simulink model "ScriptDemo"  (R2022b)
settings: configuration reference "TmVcThermal_Configuration_sub" (kept outside this file)
undefined symbols (not defined in the file or in its folder): aaaa, bbbb, cTmComprCtrl_D_u8HvacFlowTable_db, cTmComprCtrl_D_u8HvacFlowTable_sw, cTmComprCtrl_n_i16ChillCmpIMax, cTmComprCtrl_n_i16ChillCmpIMin, cTmComprCtrl_n_i16ChillCmpIMin666, cTmComprCtrl_n_i16ChillCmpPMax, cTmComprCtrl_n_i16ChillCmpPMin, cTmComprCtrl_n_i16CmpChillCoolRpmKiMax, cTmComprCtrl_n_i16CmpChillCoolRpmKiMin, cTmComprCtrl_n_i16CmpChillCoolRpmKpMax, cTmComprCtrl_n_i16CmpChillCoolRpmKpMin, cTmComprCtrl_n_i16CmpCoolRpmKiMax, cTmComprCtrl_n_i16CmpCoolRpmKiMin, cTmComprCtrl_n_i16CmpCoolRpmKpMax, cTmComprCtrl_n_i16CmpCoolRpmKpMin, cTmComprCtrl_n_i16SM4CmpHeatKiMax, cTmComprCtrl_n_i16SM4CmpHeatKiMin, cTmComprCtrl_n_i16SM4CmpHeatKpMax, cTmComprCtrl_n_i16SM4CmpHeatKpMin, cTmComprCtrl_n_i16SM5CmpHeatKiMax, cTmComprCtrl_n_i16SM5CmpHeatKiMin, cTmComprCtrl_n_i16SM5CmpHeatKpMax, cTmComprCtrl_n_i16SM5CmpHeatKpMin, cTmComprCtrl_n_i16SM6CmpHeatKiMax, cTmComprCtrl_n_i16SM6CmpHeatKiMin, cTmComprCtrl_n_i16SM6CmpHeatKpMax, cTmComprCtrl_n_i16SM6CmpHeatKpMin, cTmComprCtrl_n_u16CmpMaxSpdFanFltLimt, cTmComprCtrl_n_u16CmpMaxSpdLoSidePFltLimt, cTmComprCtrl_n_u16CmpMaxSpdSensorFltLimt, cTmComprCtrl_n_u16CompMinRpm, cTmComprCtrl_n_u16CompRpmIncThres, cTmComprCtrl_t_u16BattCooltFFPeriod, cTmComprCtrl_t_u16BattCooltPIPeriod, cTmComprCtrl_t_u16CmpCoolFFPeriod, cTmComprCtrl_t_u16CmpCoolPIPeriod, cTmComprCtrl_t_u16CoolCmpChillFFPeriod, cTmComprCtrl_t_u16CoolCmpChillPIPeriod, cTmComprCtrl_t_u16SM4CmpHeatFFPeriod, cTmComprCtrl_t_u16SM4CmpHeatPIPeriod, cTmComprCtrl_t_u16SM5CmpHeatFFPeriod, cTmComprCtrl_t_u16SM5CmpHeatPIPeriod, cTmComprCtrl_t_u16SM6CmpHeatFFPeriod, cTmComprCtrl_t_u16SM6CmpHeatPIPeriod, cTmComprCtrl_Te_EvapClearInteg, cTmComprCtrl_Te_i16HpReqTempSaturoffset, cTmComprCtrl_Te_i16SatLpReplaceDiff, cTmComprCtrl_Te_i16SM3BatDiffStartEvapDecOffset, cTmComprCtrl_Te_i16SM3EvapLo, cTmComprCtrl_Te_i16SM3TBatDiffEntEvapDecOffset, cTmComprCtrl_Te_i16SM3TBatDiffEntEvapDecOffsetQuit, cTmComprCtrl_Te_s32ErrCmpChillPIContinueCoolH, cTmComprCtrl_Te_s32ErrCmpChillPIContinueCoolL, cTmComprCtrl_Te_s32ErrCmpPIContinueChillH, cTmComprCtrl_Te_s32ErrCmpPIContinueChillL, cTmComprCtrl_Te_s32ErrCmpPIContinueCoolH, cTmComprCtrl_Te_s32ErrCmpPIContinueCoolL, cTmComprCtrl_Te_s32ErrCmpPIContinueHeatH ... (+398)
libraries: simulink x846, PCMULib x711, simulink_need_slupdate x4
(part 8 of 49)

== system ScriptDemo/Create/creatTmBaseArch/Before ==

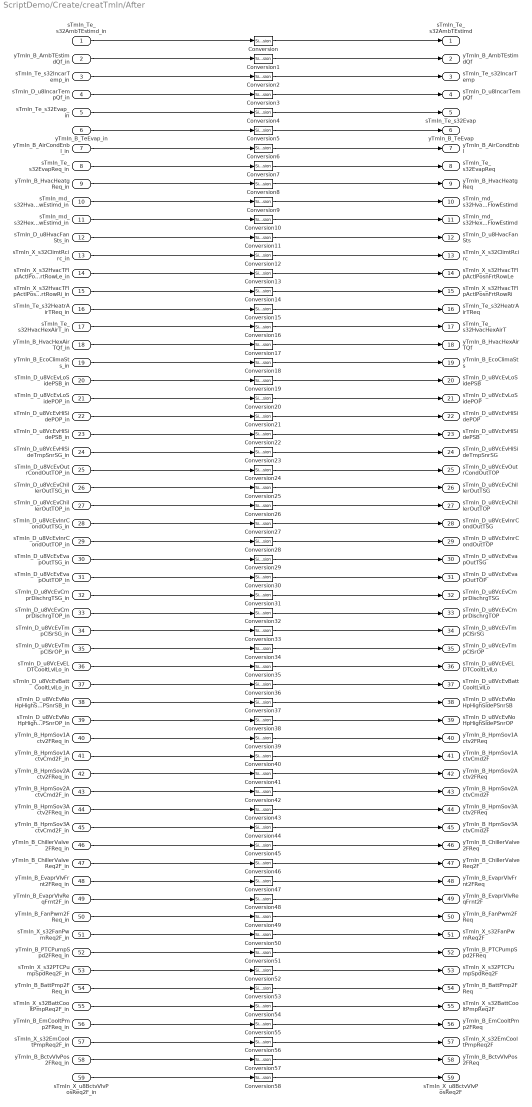
== system ScriptDemo/Create/creatTmIn/After ==
  sTmIn_Te_s32AmbTEstimd_in : Inport
  yTmIn_B_AmbTEstimdQf_in : Inport  Port=2
  sTmIn_Te_s32IncarTemp_in : Inport  Port=3
  sTmIn_D_u8IncarTempQf_in : Inport  Port=4
  sTmIn_Te_s32Evap_in : Inport  Port=5
  yTmIn_B_TeEvap_in : Inport  Port=6
  yTmIn_B_AirCondEnbl_in : Inport  Port=7
  sTmIn_Te_s32EvapReq_in : Inport  Port=8
  yTmIn_B_HvacHeatgReq_in : Inport  Port=9
  sTmIn_md_s32HvacAirMFlowEstimd_in : Inport  Port=10
  sTmIn_md_s32HexHeatrAirMFlowEstimd_in : Inport  Port=11
  sTmIn_D_u8HvacFanSts_in : Inport  Port=12
  sTmIn_X_s32ClimtRcirc_in : Inport  Port=13
  sTmIn_X_s32HvacTFlpActlPosnFrtRowLe_in : Inport  Port=14
  sTmIn_X_s32HvacTFlpActlPosnFrtRowRi_in : Inport  Port=15
  sTmIn_Te_s32HeatrAirTReq_in : Inport  Port=16
  sTmIn_Te_s32HvacHexAirT_in : Inport  Port=17
  yTmIn_B_HvacHexAirTQf_in : Inport  Port=18
  yTmIn_B_EcoClimaSts_in : Inport  Port=19
  sTmIn_D_u8VcEvLoSidePSB_in : Inport  Port=20
  sTmIn_D_u8VcEvLoSidePOP_in : Inport  Port=21
  sTmIn_D_u8VcEvHiSidePOP_in : Inport  Port=22
  sTmIn_D_u8VcEvHiSidePSB_in : Inport  Port=23
  sTmIn_D_u8VcEvHiSideTmpSnrSG_in : Inport  Port=24
  sTmIn_D_u8VcEvOutrCondOutTOP_in : Inport  Port=25
  sTmIn_D_u8VcEvChillerOutTSG_in : Inport  Port=26
  sTmIn_D_u8VcEvChillerOutTOP_in : Inport  Port=27
  sTmIn_D_u8VcEvInrCondOutTSG_in : Inport  Port=28
  sTmIn_D_u8VcEvInrCondOutTOP_in : Inport  Port=29
  sTmIn_D_u8VcEvEvapOutTSG_in : Inport  Port=30
  sTmIn_D_u8VcEvEvapOutTOP_in : Inport  Port=31
  sTmIn_D_u8VcEvCmprDischrgTSG_in : Inport  Port=32
  sTmIn_D_u8VcEvCmprDischrgTOP_in : Inport  Port=33
  sTmIn_D_u8VcEvTmpClSrSG_in : Inport  Port=34
  sTmIn_D_u8VcEvTmpClSrOP_in : Inport  Port=35
  sTmIn_D_u8VcEvELDTCooltLvlLo_in : Inport  Port=36
  sTmIn_D_u8VcEvBattCooltLvlLo_in : Inport  Port=37
  sTmIn_D_u8VcEvNoHpHighSidePSnrSB_in : Inport  Port=38
  sTmIn_D_u8VcEvNoHpHighSidePSnrOP_in : Inport  Port=39
  yTmIn_B_HpmSov1Actv2FReq_in : Inport  Port=40
  yTmIn_B_HpmSov1ActvCmd2F_in : Inport  Port=41
  yTmIn_B_HpmSov2Actv2FReq_in : Inport  Port=42
  yTmIn_B_HpmSov2ActvCmd2F_in : Inport  Port=43
  yTmIn_B_HpmSov3Actv2FReq_in : Inport  Port=44
  yTmIn_B_HpmSov3ActvCmd2F_in : Inport  Port=45
  yTmIn_B_ChillerValve2FReq_in : Inport  Port=46
  yTmIn_B_ChillerValveReq2F_in : Inport  Port=47
  yTmIn_B_EvaprVlvFrnt2FReq_in : Inport  Port=48
  yTmIn_B_EvaprVlvReqFrnt2F_in : Inport  Port=49
  yTmIn_B_FanPwm2FReq_in : Inport  Port=50
  sTmIn_X_s32FanPwmReq2F_in : Inport  Port=51
  yTmIn_B_PTCPumpSpd2FReq_in : Inport  Port=52
  sTmIn_X_s32PTCPumpSpdReq2F_in : Inport  Port=53
  yTmIn_B_BattPmp2FReq_in : Inport  Port=54
  sTmIn_X_s32BattCooltPmpReq2F_in : Inport  Port=55
  yTmIn_B_EmCooltPmp2FReq_in : Inport  Port=56
  sTmIn_X_s32EmCooltPmpReq2F_in : Inport  Port=57
  yTmIn_B_BctvVlvPos2FReq_in : Inport  Port=58
  sTmIn_X_u8BctvVlvPosReq2F_in : Inport  Port=59
  Conversion{,1..58} (59 alike) : SignalConversion  OverrideOpt=off
  sTmIn_Te_s32AmbTEstimd : Outport
  yTmIn_B_AmbTEstimdQf : Outport  Port=2
  sTmIn_Te_s32IncarTemp : Outport  Port=3
  sTmIn_D_u8IncarTempQf : Outport  Port=4
  sTmIn_Te_s32Evap : Outport  Port=5
  yTmIn_B_TeEvap : Outport  Port=6
  yTmIn_B_AirCondEnbl : Outport  Port=7
  sTmIn_Te_s32EvapReq : Outport  Port=8
  yTmIn_B_HvacHeatgReq : Outport  Port=9
  sTmIn_md_s32HvacAirMFlowEstimd : Outport  Port=10
  sTmIn_md_s32HexHeatrAirMFlowEstimd : Outport  Port=11
  sTmIn_D_u8HvacFanSts : Outport  Port=12
  sTmIn_X_s32ClimtRcirc : Outport  Port=13
  sTmIn_X_s32HvacTFlpActlPosnFrtRowLe : Outport  Port=14
  sTmIn_X_s32HvacTFlpActlPosnFrtRowRi : Outport  Port=15
  sTmIn_Te_s32HeatrAirTReq : Outport  Port=16
  sTmIn_Te_s32HvacHexAirT : Outport  Port=17
  yTmIn_B_HvacHexAirTQf : Outport  Port=18
  yTmIn_B_EcoClimaSts : Outport  Port=19
  sTmIn_D_u8VcEvLoSidePSB : Outport  Port=20
  sTmIn_D_u8VcEvLoSidePOP : Outport  Port=21
  sTmIn_D_u8VcEvHiSidePOP : Outport  Port=22
  sTmIn_D_u8VcEvHiSidePSB : Outport  Port=23
  sTmIn_D_u8VcEvHiSideTmpSnrSG : Outport  Port=24
  sTmIn_D_u8VcEvOutrCondOutTOP : Outport  Port=25
  sTmIn_D_u8VcEvChillerOutTSG : Outport  Port=26
  sTmIn_D_u8VcEvChillerOutTOP : Outport  Port=27
  sTmIn_D_u8VcEvInrCondOutTSG : Outport  Port=28
  sTmIn_D_u8VcEvInrCondOutTOP : Outport  Port=29
  sTmIn_D_u8VcEvEvapOutTSG : Outport  Port=30
  sTmIn_D_u8VcEvEvapOutTOP : Outport  Port=31
  sTmIn_D_u8VcEvCmprDischrgTSG : Outport  Port=32
  sTmIn_D_u8VcEvCmprDischrgTOP : Outport  Port=33
  sTmIn_D_u8VcEvTmpClSrSG : Outport  Port=34
  sTmIn_D_u8VcEvTmpClSrOP : Outport  Port=35
  sTmIn_D_u8VcEvELDTCooltLvlLo : Outport  Port=36
  sTmIn_D_u8VcEvBattCooltLvlLo : Outport  Port=37
  sTmIn_D_u8VcEvNoHpHighSidePSnrSB : Outport  Port=38
  sTmIn_D_u8VcEvNoHpHighSidePSnrOP : Outport  Port=39
  yTmIn_B_HpmSov1Actv2FReq : Outport  Port=40
  yTmIn_B_HpmSov1ActvCmd2F : Outport  Port=41
  yTmIn_B_HpmSov2Actv2FReq : Outport  Port=42
  yTmIn_B_HpmSov2ActvCmd2F : Outport  Port=43
  yTmIn_B_HpmSov3Actv2FReq : Outport  Port=44
  yTmIn_B_HpmSov3ActvCmd2F : Outport  Port=45
  yTmIn_B_ChillerValve2FReq : Outport  Port=46
  yTmIn_B_ChillerValveReq2F : Outport  Port=47
  yTmIn_B_EvaprVlvFrnt2FReq : Outport  Port=48
  yTmIn_B_EvaprVlvReqFrnt2F : Outport  Port=49
  yTmIn_B_FanPwm2FReq : Outport  Port=50
  sTmIn_X_s32FanPwmReq2F : Outport  Port=51
  yTmIn_B_PTCPumpSpd2FReq : Outport  Port=52
  sTmIn_X_s32PTCPumpSpdReq2F : Outport  Port=53
  yTmIn_B_BattPmp2FReq : Outport  Port=54
  sTmIn_X_s32BattCooltPmpReq2F : Outport  Port=55
  yTmIn_B_EmCooltPmp2FReq : Outport  Port=56
  sTmIn_X_s32EmCooltPmpReq2F : Outport  Port=57
  yTmIn_B_BctvVlvPos2FReq : Outport  Port=58
  sTmIn_X_u8BctvVlvPosReq2F : Outport  Port=59
  wires:
  Conversion54/1 -> sTmIn_X_s32BattCooltPmpReq2F/1
  Conversion53/1 -> yTmIn_B_BattPmp2FReq/1
  yTmIn_B_HpmSov2ActvCmd2F_in/1 -> Conversion42/1
  yTmIn_B_ChillerValve2FReq_in/1 -> Conversion45/1
  Conversion19/1 -> sTmIn_D_u8VcEvLoSidePSB/1
  yTmIn_B_HpmSov3ActvCmd2F_in/1 -> Conversion44/1
  sTmIn_X_s32EmCooltPmpReq2F_in/1 -> Conversion56/1
  Conversion8/1 -> yTmIn_B_HvacHeatgReq/1
  yTmIn_B_HvacHeatgReq_in/1 -> Conversion8/1
  Conversion43/1 -> yTmIn_B_HpmSov3Actv2FReq/1
  Conversion6/1 -> yTmIn_B_AirCondEnbl/1
  sTmIn_D_u8VcEvInrCondOutTOP_in/1 -> Conversion28/1
  Conversion1/1 -> yTmIn_B_AmbTEstimdQf/1
  yTmIn_B_BctvVlvPos2FReq_in/1 -> Conversion57/1
  Conversion56/1 -> sTmIn_X_s32EmCooltPmpReq2F/1
  yTmIn_B_AirCondEnbl_in/1 -> Conversion6/1
  sTmIn_D_u8VcEvBattCooltLvlLo_in/1 -> Conversion36/1
  yTmIn_B_AmbTEstimdQf_in/1 -> Conversion1/1
  yTmIn_B_HpmSov1ActvCmd2F_in/1 -> Conversion40/1
  yTmIn_B_PTCPumpSpd2FReq_in/1 -> Conversion51/1
  yTmIn_B_HpmSov2Actv2FReq_in/1 -> Conversion41/1
  Conversion34/1 -> sTmIn_D_u8VcEvTmpClSrOP/1
  Conversion32/1 -> sTmIn_D_u8VcEvCmprDischrgTOP/1
  Conversion17/1 -> yTmIn_B_HvacHexAirTQf/1
  Conversion24/1 -> sTmIn_D_u8VcEvOutrCondOutTOP/1
  Conversion40/1 -> yTmIn_B_HpmSov1ActvCmd2F/1
  Conversion41/1 -> yTmIn_B_HpmSov2Actv2FReq/1
  Conversion55/1 -> yTmIn_B_EmCooltPmp2FReq/1
  sTmIn_Te_s32EvapReq_in/1 -> Conversion7/1
  sTmIn_D_u8VcEvEvapOutTOP_in/1 -> Conversion30/1
  Conversion39/1 -> yTmIn_B_HpmSov1Actv2FReq/1
  sTmIn_X_s32ClimtRcirc_in/1 -> Conversion12/1
  Conversion14/1 -> sTmIn_X_s32HvacTFlpActlPosnFrtRowRi/1
  sTmIn_Te_s32Evap_in/1 -> Conversion4/1
  Conversion58/1 -> sTmIn_X_u8BctvVlvPosReq2F/1
  Conversion42/1 -> yTmIn_B_HpmSov2ActvCmd2F/1
  sTmIn_D_u8IncarTempQf_in/1 -> Conversion3/1
  Conversion57/1 -> yTmIn_B_BctvVlvPos2FReq/1
  yTmIn_B_BattPmp2FReq_in/1 -> Conversion53/1
  sTmIn_X_s32BattCooltPmpReq2F_in/1 -> Conversion54/1
  yTmIn_B_EmCooltPmp2FReq_in/1 -> Conversion55/1
  sTmIn_D_u8VcEvEvapOutTSG_in/1 -> Conversion29/1
  Conversion/1 -> sTmIn_Te_s32AmbTEstimd/1
  sTmIn_X_s32HvacTFlpActlPosnFrtRowRi_in/1 -> Conversion14/1
  sTmIn_D_u8VcEvELDTCooltLvlLo_in/1 -> Conversion35/1
  Conversion35/1 -> sTmIn_D_u8VcEvELDTCooltLvlLo/1
  Conversion44/1 -> yTmIn_B_HpmSov3ActvCmd2F/1
  Conversion38/1 -> sTmIn_D_u8VcEvNoHpHighSidePSnrOP/1
  Conversion3/1 -> sTmIn_D_u8IncarTempQf/1
  Conversion30/1 -> sTmIn_D_u8VcEvEvapOutTOP/1
  Conversion4/1 -> sTmIn_Te_s32Evap/1
  Conversion23/1 -> sTmIn_D_u8VcEvHiSideTmpSnrSG/1
  Conversion25/1 -> sTmIn_D_u8VcEvChillerOutTSG/1
  Conversion7/1 -> sTmIn_Te_s32EvapReq/1
  Conversion33/1 -> sTmIn_D_u8VcEvTmpClSrSG/1
  yTmIn_B_HpmSov3Actv2FReq_in/1 -> Conversion43/1
  Conversion36/1 -> sTmIn_D_u8VcEvBattCooltLvlLo/1
  yTmIn_B_HpmSov1Actv2FReq_in/1 -> Conversion39/1
  sTmIn_D_u8VcEvCmprDischrgTOP_in/1 -> Conversion32/1
  Conversion29/1 -> sTmIn_D_u8VcEvEvapOutTSG/1
  sTmIn_D_u8VcEvNoHpHighSidePSnrOP_in/1 -> Conversion38/1
  Conversion11/1 -> sTmIn_D_u8HvacFanSts/1
  sTmIn_Te_s32IncarTemp_in/1 -> Conversion2/1
  Conversion2/1 -> sTmIn_Te_s32IncarTemp/1
  sTmIn_D_u8VcEvTmpClSrSG_in/1 -> Conversion33/1
  yTmIn_B_ChillerValveReq2F_in/1 -> Conversion46/1
  yTmIn_B_FanPwm2FReq_in/1 -> Conversion49/1
  sTmIn_D_u8VcEvTmpClSrOP_in/1 -> Conversion34/1
  sTmIn_D_u8VcEvCmprDischrgTSG_in/1 -> Conversion31/1
  Conversion31/1 -> sTmIn_D_u8VcEvCmprDischrgTSG/1
  yTmIn_B_TeEvap_in/1 -> Conversion5/1
  Conversion5/1 -> yTmIn_B_TeEvap/1
  sTmIn_Te_s32AmbTEstimd_in/1 -> Conversion/1
  Conversion37/1 -> sTmIn_D_u8VcEvNoHpHighSidePSnrSB/1
  sTmIn_D_u8VcEvNoHpHighSidePSnrSB_in/1 -> Conversion37/1
  Conversion49/1 -> yTmIn_B_FanPwm2FReq/1
  sTmIn_X_s32FanPwmReq2F_in/1 -> Conversion50/1
  Conversion50/1 -> sTmIn_X_s32FanPwmReq2F/1
  Conversion15/1 -> sTmIn_Te_s32HeatrAirTReq/1
  Conversion51/1 -> yTmIn_B_PTCPumpSpd2FReq/1
  sTmIn_X_s32PTCPumpSpdReq2F_in/1 -> Conversion52/1
  Conversion52/1 -> sTmIn_X_s32PTCPumpSpdReq2F/1
  yTmIn_B_EvaprVlvReqFrnt2F_in/1 -> Conversion48/1
  Conversion13/1 -> sTmIn_X_s32HvacTFlpActlPosnFrtRowLe/1
  Conversion48/1 -> yTmIn_B_EvaprVlvReqFrnt2F/1
  Conversion9/1 -> sTmIn_md_s32HvacAirMFlowEstimd/1
  sTmIn_md_s32HexHeatrAirMFlowEstimd_in/1 -> Conversion10/1
  sTmIn_D_u8VcEvLoSidePOP_in/1 -> Conversion20/1
  sTmIn_D_u8VcEvChillerOutTOP_in/1 -> Conversion26/1
  Conversion10/1 -> sTmIn_md_s32HexHeatrAirMFlowEstimd/1
  Conversion18/1 -> yTmIn_B_EcoClimaSts/1
  sTmIn_D_u8HvacFanSts_in/1 -> Conversion11/1
  sTmIn_md_s32HvacAirMFlowEstimd_in/1 -> Conversion9/1
  sTmIn_Te_s32HvacHexAirT_in/1 -> Conversion16/1
  Conversion16/1 -> sTmIn_Te_s32HvacHexAirT/1
  yTmIn_B_HvacHexAirTQf_in/1 -> Conversion17/1
  yTmIn_B_EcoClimaSts_in/1 -> Conversion18/1
  Conversion26/1 -> sTmIn_D_u8VcEvChillerOutTOP/1
  sTmIn_D_u8VcEvHiSidePOP_in/1 -> Conversion21/1
  Conversion21/1 -> sTmIn_D_u8VcEvHiSidePOP/1
  sTmIn_D_u8VcEvHiSidePSB_in/1 -> Conversion22/1
  Conversion27/1 -> sTmIn_D_u8VcEvInrCondOutTSG/1
  Conversion47/1 -> yTmIn_B_EvaprVlvFrnt2FReq/1
  Conversion22/1 -> sTmIn_D_u8VcEvHiSidePSB/1
  sTmIn_D_u8VcEvHiSideTmpSnrSG_in/1 -> Conversion23/1
  sTmIn_D_u8VcEvOutrCondOutTOP_in/1 -> Conversion24/1
  sTmIn_D_u8VcEvChillerOutTSG_in/1 -> Conversion25/1
  sTmIn_Te_s32HeatrAirTReq_in/1 -> Conversion15/1
  Conversion46/1 -> yTmIn_B_ChillerValveReq2F/1
  yTmIn_B_EvaprVlvFrnt2FReq_in/1 -> Conversion47/1
  Conversion45/1 -> yTmIn_B_ChillerValve2FReq/1
  sTmIn_X_u8BctvVlvPosReq2F_in/1 -> Conversion58/1
  Conversion28/1 -> sTmIn_D_u8VcEvInrCondOutTOP/1
  sTmIn_D_u8VcEvInrCondOutTSG_in/1 -> Conversion27/1
  Conversion20/1 -> sTmIn_D_u8VcEvLoSidePOP/1
  Conversion12/1 -> sTmIn_X_s32ClimtRcirc/1
  sTmIn_X_s32HvacTFlpActlPosnFrtRowLe_in/1 -> Conversion13/1
  sTmIn_D_u8VcEvLoSidePSB_in/1 -> Conversion19/1

== system ScriptDemo/Create/creatTmIn/Before ==

== system ScriptDemo/Create/creatTmOut/Before ==
  TmBase2Out : Subsystem
  wires:
  [sTmComprCtrl_n_u16CompRpmReq] -> TmBase2Out/1(sTmComprCtrl_n_u16CompRpmReq)
  [yTmComprCtrl_B_CompOnReq] -> TmBase2Out/2(yTmComprCtrl_B_CompOnReq)
  [sTmEnergyMgr_Pw_s32AcCmprPwrLim] -> TmBase2Out/3(sTmEnergyMgr_Pw_s32AcCmprPwrLim)
  [sTmRefriVlvCtrl_X_s32EEXVPosReq] -> TmBase2Out/4(sTmRefriVlvCtrl_X_s32EEXVPosReq)
  [yTmRefriVlvCtrl_B_EexvCalibReq] -> TmBase2Out/5(yTmRefriVlvCtrl_B_EexvCalibReq)
  [yTmRefriVlvCtrl_B_HpcEexvMovEnable] -> TmBase2Out/6(yTmRefriVlvCtrl_B_HpcEexvMovEnable)
  [sTmRefriVlvCtrl_X_s32BEXVPosReq] -> TmBase2Out/7(sTmRefriVlvCtrl_X_s32BEXVPosReq)
  [yTmRefriVlvCtrl_B_BexvCalibReq] -> TmBase2Out/8(yTmRefriVlvCtrl_B_BexvCalibReq)
  [yTmRefriVlvCtrl_B_HpcBexvMovEnable] -> TmBase2Out/9(yTmRefriVlvCtrl_B_HpcBexvMovEnable)
  [sTmRefriVlvCtrl_X_s32CEXVPosReq] -> TmBase2Out/10(sTmRefriVlvCtrl_X_s32CEXVPosReq)
  [yTmRefriVlvCtrl_B_CexvCalibReq] -> TmBase2Out/11(yTmRefriVlvCtrl_B_CexvCalibReq)
  [yTmRefriVlvCtrl_B_HpcCexvMovEnable] -> TmBase2Out/12(yTmRefriVlvCtrl_B_HpcCexvMovEnable)
  [sTmColtVlvCtrl_D_u8HpcBctvRefDrvReq] -> TmBase2Out/13(sTmColtVlvCtrl_D_u8HpcBctvRefDrvReq)
  [sTmColtVlvCtrl_X_u8BctvPosReq] -> TmBase2Out/14(sTmColtVlvCtrl_X_u8BctvPosReq)
  [sTmColtVlvCtrl_D_u8HpcBcfvRefDrvReq] -> TmBase2Out/15(sTmColtVlvCtrl_D_u8HpcBcfvRefDrvReq)
  [sTmDiag_D_u8VcEvLowSidePSnrSB] -> TmBase2Out/16(sTmDiag_D_u8VcEvLowSidePSnrSB)
  [sTmDiag_D_u8VcEvLowSidePSnrOP] -> TmBase2Out/17(sTmDiag_D_u8VcEvLowSidePSnrOP)
  [sTmDiag_D_u8VcEvHiSidePSnrOP] -> TmBase2Out/18(sTmDiag_D_u8VcEvHiSidePSnrOP)
  [sTmDiag_D_u8VcEvHiSidePSnrSB] -> TmBase2Out/19(sTmDiag_D_u8VcEvHiSidePSnrSB)
  [sTmDiag_D_u8VcEvHiSideTmpSnrSG] -> TmBase2Out/20(sTmDiag_D_u8VcEvHiSideTmpSnrSG)
  [sTmDiag_D_u8VcEvHiSideTmpSnrOP] -> TmBase2Out/21(sTmDiag_D_u8VcEvHiSideTmpSnrOP)
  [sTmDiag_D_u8VcEvBattCooltLvlLo] -> TmBase2Out/22(sTmDiag_D_u8VcEvBattCooltLvlLo)
  [sTmDiag_D_u8VcEvSov1SB] -> TmBase2Out/23(sTmDiag_D_u8VcEvSov1SB)
  [sTmDiag_D_u8VcEvSov2SB] -> TmBase2Out/24(sTmDiag_D_u8VcEvSov2SB)
  [sTmDiag_D_u8VcEvSov3SB] -> TmBase2Out/25(sTmDiag_D_u8VcEvSov3SB)
  [sTmDiag_D_u8VcEvSov5SB] -> TmBase2Out/26(sTmDiag_D_u8VcEvSov5SB)
  [sTmDiag_D_u8VcEvSov4SB] -> TmBase2Out/27(sTmDiag_D_u8VcEvSov4SB)
  [sTmDiag_D_u8VcEvSBFan] -> TmBase2Out/28(sTmDiag_D_u8VcEvSBFan)
  [sTmDiag_D_u8VcEvOPFan] -> TmBase2Out/29(sTmDiag_D_u8VcEvOPFan)
  [sTmDiag_D_u8VcEvSGFan] -> TmBase2Out/30(sTmDiag_D_u8VcEvSGFan)
  [sTmDiag_D_u8VcEvVolErrFan] -> TmBase2Out/31(sTmDiag_D_u8VcEvVolErrFan)
  [sTmDiag_D_u8VcEvBlokFan] -> TmBase2Out/32(sTmDiag_D_u8VcEvBlokFan)
  [sTmDiag_D_u8VcEvCircutInteFlt] -> TmBase2Out/33(sTmDiag_D_u8VcEvCircutInteFlt)
  [sTmDiag_D_u8VcEvHmPumpSB] -> TmBase2Out/34(sTmDiag_D_u8VcEvHmPumpSB)
  [sTmDiag_D_u8VcEvHmPumpOC] -> TmBase2Out/35(sTmDiag_D_u8VcEvHmPumpOC)
  [sTmDiag_D_u8HpmSov1Actv2FEnState] -> TmBase2Out/36(sTmDiag_D_u8HpmSov1Actv2FEnState)
  [sTmDiag_D_u8HpmSov2Actv2FEnState] -> TmBase2Out/37(sTmDiag_D_u8HpmSov2Actv2FEnState)
  [sTmDiag_D_u8HpmSov3Actv2FEnState] -> TmBase2Out/38(sTmDiag_D_u8HpmSov3Actv2FEnState)
  [sTmDiag_D_u8FanPwm2FEnState] -> TmBase2Out/39(sTmDiag_D_u8FanPwm2FEnState)
  [sTmDiag_D_u8BattCooltPmp2FEnState] -> TmBase2Out/40(sTmDiag_D_u8BattCooltPmp2FEnState)
  [sTmDiag_D_u8EmCooltPmp2FEnState] -> TmBase2Out/41(sTmDiag_D_u8EmCooltPmp2FEnState)
  [sTmDiag_D_u8PTCPumpSpd2FEnState] -> TmBase2Out/42(sTmDiag_D_u8PTCPumpSpd2FEnState)
  [sTmDiag_D_u8EctvVlvMoveEna2FEnaState] -> TmBase2Out/43(sTmDiag_D_u8EctvVlvMoveEna2FEnaState)
  [sTmDiag_D_u8EctvVlvPos2FEnaState] -> TmBase2Out/44(sTmDiag_D_u8EctvVlvPos2FEnaState)
  [sTmDiag_D_u8BctvVlvRef2FEnaState] -> TmBase2Out/45(sTmDiag_D_u8BctvVlvRef2FEnaState)
  [sTmDiag_D_u8BctvVlvPos2FEnaState] -> TmBase2Out/46(sTmDiag_D_u8BctvVlvPos2FEnaState)
  [sTmDiag_D_u8BcfvVlvRef2FEnaState] -> TmBase2Out/47(sTmDiag_D_u8BcfvVlvRef2FEnaState)
  [sTmDiag_D_u8BcfvVlvPos2FEnaState] -> TmBase2Out/48(sTmDiag_D_u8BcfvVlvPos2FEnaState)
  [sTmDiag_D_u8BexvCal2FEnaState] -> TmBase2Out/49(sTmDiag_D_u8BexvCal2FEnaState)
  [sTmDiag_D_u8BexvMoveEna2FEnaState] -> TmBase2Out/50(sTmDiag_D_u8BexvMoveEna2FEnaState)
  [sTmDiag_D_u8BexvPosnReq2FEnaState] -> TmBase2Out/51(sTmDiag_D_u8BexvPosnReq2FEnaState)
  [sTmDiag_D_u8CexvCal2FEnaState] -> TmBase2Out/52(sTmDiag_D_u8CexvCal2FEnaState)
  [sTmDiag_D_u8CexvMoveEna2FEnaState] -> TmBase2Out/53(sTmDiag_D_u8CexvMoveEna2FEnaState)
  [sTmDiag_D_u8CexvPosnReq2FEnaState] -> TmBase2Out/54(sTmDiag_D_u8CexvPosnReq2FEnaState)
  [sTmDiag_D_u8EexvCal2FEnaState] -> TmBase2Out/55(sTmDiag_D_u8EexvCal2FEnaState)
  TmBase2Out/1(sTmOut_n_u16ElacCmprReq) -> [sTmOut_n_u16ElacCmprReq]
  TmBase2Out/2(sTmOut_D_u8ElacCmprRelease) -> [sTmOut_D_u8ElacCmprRelease]
  TmBase2Out/3(sTmOut_Pw_s32ElacCmprMax) -> [sTmOut_Pw_s32ElacCmprMax]
  TmBase2Out/4(sTmOut_X_s32EexvVlvPosReq) -> [sTmOut_X_s32EexvVlvPosReq]
  TmBase2Out/5(yTmOut_B_EexvPosnCalibReq) -> [yTmOut_B_EexvPosnCalibReq]
  TmBase2Out/6(yTmOut_B_EexvPosnMovEnable) -> [yTmOut_B_EexvPosnMovEnable]
  TmBase2Out/7(sTmOut_X_s32BexvVlvPosReq) -> [sTmOut_X_s32BexvVlvPosReq]
  TmBase2Out/8(yTmOut_B_BexvPosnCalibReq) -> [yTmOut_B_BexvPosnCalibReq]
  TmBase2Out/9(yTmOut_B_BexvPosnMovEnable) -> [yTmOut_B_BexvPosnMovEnable]
  TmBase2Out/10(sTmOut_X_s32CexvVlvPosReq) -> [sTmOut_X_s32CexvVlvPosReq]
  TmBase2Out/11(yTmOut_B_CexvPosnCalibReq) -> [yTmOut_B_CexvPosnCalibReq]
  TmBase2Out/12(yTmOut_B_CexvPosnMovEnable) -> [yTmOut_B_CexvPosnMovEnable]
  TmBase2Out/13(sTmOut_D_u8BctvVlvRefDrvReq) -> [sTmOut_D_u8BctvVlvRefDrvReq]
  TmBase2Out/14(sTmOut_X_u8BctvVlvPosReq) -> [sTmOut_X_u8BctvVlvPosReq]
  TmBase2Out/15(sTmOut_D_u8BcfvVlvRefDrvReq) -> [sTmOut_D_u8BcfvVlvRefDrvReq]
  TmBase2Out/16(sTmOut_D_u8VcEvLowSidePSnrSB) -> [sTmOut_D_u8VcEvLowSidePSnrSB]
  TmBase2Out/17(sTmOut_D_u8VcEvLowSidePSnrOP) -> [sTmOut_D_u8VcEvLowSidePSnrOP]
  TmBase2Out/18(sTmOut_D_u8VcEvHiSidePSnrOP) -> [sTmOut_D_u8VcEvHiSidePSnrOP]
  TmBase2Out/19(sTmOut_D_u8VcEvHiSidePSnrSB) -> [sTmOut_D_u8VcEvHiSidePSnrSB]
  TmBase2Out/20(sTmOut_D_u8VcEvHiSideTmpSnrSG) -> [sTmOut_D_u8VcEvHiSideTmpSnrSG]
  TmBase2Out/21(sTmOut_D_u8VcEvHiSideTmpSnrOP) -> [sTmOut_D_u8VcEvHiSideTmpSnrOP]
  TmBase2Out/22(sTmOut_D_u8VcEvBattCooltLvlLo) -> [sTmOut_D_u8VcEvBattCooltLvlLo]
  TmBase2Out/23(sTmOut_D_u8VcEvSov1SB) -> [sTmOut_D_u8VcEvSov1SB]
  TmBase2Out/24(sTmOut_D_u8VcEvSov2SB) -> [sTmOut_D_u8VcEvSov2SB]
  TmBase2Out/25(sTmOut_D_u8VcEvSov3SB) -> [sTmOut_D_u8VcEvSov3SB]
  TmBase2Out/26(sTmOut_D_u8VcEvSov5SB) -> [sTmOut_D_u8VcEvSov5SB]
  TmBase2Out/27(sTmOut_D_u8VcEvSov4SB) -> [sTmOut_D_u8VcEvSov4SB]
  TmBase2Out/28(sTmOut_D_u8VcEvSBFan) -> [sTmOut_D_u8VcEvSBFan]
  TmBase2Out/29(sTmOut_D_u8VcEvOPFan) -> [sTmOut_D_u8VcEvOPFan]
  TmBase2Out/30(sTmOut_D_u8VcEvSGFan) -> [sTmOut_D_u8VcEvSGFan]
  TmBase2Out/31(sTmOut_D_u8VcEvVolErrFan) -> [sTmOut_D_u8VcEvVolErrFan]
  TmBase2Out/32(sTmOut_D_u8VcEvBlokFan) -> [sTmOut_D_u8VcEvBlokFan]
  TmBase2Out/33(sTmOut_D_u8VcEvCircutInteFlt) -> [sTmOut_D_u8VcEvCircutInteFlt]
  TmBase2Out/34(sTmOut_D_u8VcEvHmPumpSB) -> [sTmOut_D_u8VcEvHmPumpSB]
  TmBase2Out/35(sTmOut_D_u8VcEvHmPumpOC) -> [sTmOut_D_u8VcEvHmPumpOC]
  TmBase2Out/36(sTmOut_D_u8HpmSov1Actv2FEnState) -> [sTmOut_D_u8HpmSov1Actv2FEnState]
  TmBase2Out/37(sTmOut_D_u8HpmSov2Actv2FEnState) -> [sTmOut_D_u8HpmSov2Actv2FEnState]
  TmBase2Out/38(sTmOut_D_u8HpmSov3Actv2FEnState) -> [sTmOut_D_u8HpmSov3Actv2FEnState]
  TmBase2Out/39(sTmOut_D_u8FanPwm2FEnState) -> [sTmOut_D_u8FanPwm2FEnState]
  TmBase2Out/40(sTmOut_D_u8BattCooltPmp2FEnState) -> [sTmOut_D_u8BattCooltPmp2FEnState]
  TmBase2Out/41(sTmOut_D_u8EmCooltPmp2FEnState) -> [sTmOut_D_u8EmCooltPmp2FEnState]
  TmBase2Out/42(sTmOut_D_u8PTCPumpSpd2FEnState) -> [sTmOut_D_u8PTCPumpSpd2FEnState]
  TmBase2Out/43(sTmOut_D_u8EctvVlvMoveEna2FEnaState) -> [sTmOut_D_u8EctvVlvMoveEna2FEnaState]
  TmBase2Out/44(sTmOut_D_u8EctvVlvPos2FEnaState) -> [sTmOut_D_u8EctvVlvPos2FEnaState]
  TmBase2Out/45(sTmOut_D_u8BctvVlvRef2FEnaState) -> [sTmOut_D_u8BctvVlvRef2FEnaState]
  TmBase2Out/46(sTmOut_D_u8BctvVlvPos2FEnaState) -> [sTmOut_D_u8BctvVlvPos2FEnaState]
  TmBase2Out/47(sTmOut_D_u8BcfvVlvRef2FEnaState) -> [sTmOut_D_u8BcfvVlvRef2FEnaState]
  TmBase2Out/48(sTmOut_D_u8BcfvVlvPos2FEnaState) -> [sTmOut_D_u8BcfvVlvPos2FEnaState]
  TmBase2Out/49(sTmOut_D_u8BexvCal2FEnaState) -> [sTmOut_D_u8BexvCal2FEnaState]
  TmBase2Out/50(sTmOut_D_u8BexvMoveEna2FEnaState) -> [sTmOut_D_u8BexvMoveEna2FEnaState]
  TmBase2Out/51(sTmOut_D_u8BexvPosnReq2FEnaState) -> [sTmOut_D_u8BexvPosnReq2FEnaState]
  TmBase2Out/52(sTmOut_D_u8CexvCal2FEnaState) -> [sTmOut_D_u8CexvCal2FEnaState]
  TmBase2Out/53(sTmOut_D_u8CexvMoveEna2FEnaState) -> [sTmOut_D_u8CexvMoveEna2FEnaState]
  TmBase2Out/54(sTmOut_D_u8CexvPosnReq2FEnaState) -> [sTmOut_D_u8CexvPosnReq2FEnaState]
  TmBase2Out/55(sTmOut_D_u8EexvCal2FEnaState) -> [sTmOut_D_u8EexvCal2FEnaState]

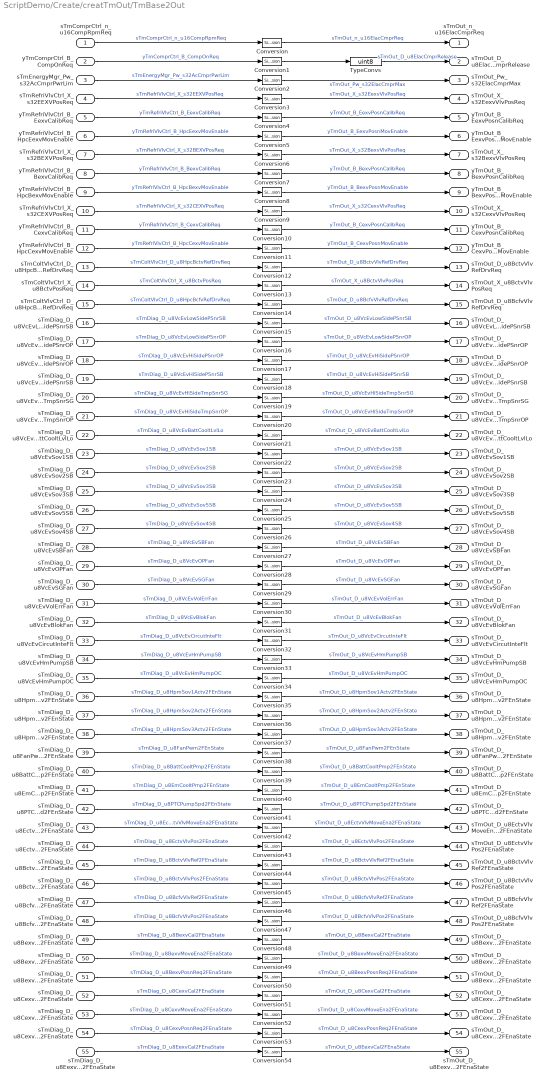
== system ScriptDemo/Create/creatTmOut/TmBase2Out ==
  sTmComprCtrl_n_u16CompRpmReq : Inport  OutDataTypeStr=uint16
  yTmComprCtrl_B_CompOnReq : Inport  Port=2  OutDataTypeStr=boolean
  sTmEnergyMgr_Pw_s32AcCmprPwrLim : Inport  Port=3  OutDataTypeStr=single
  sTmRefriVlvCtrl_X_s32EEXVPosReq : Inport  Port=4  OutDataTypeStr=single
  yTmRefriVlvCtrl_B_EexvCalibReq : Inport  Port=5  OutDataTypeStr=boolean
  yTmRefriVlvCtrl_B_HpcEexvMovEnable : Inport  Port=6  OutDataTypeStr=boolean
  sTmRefriVlvCtrl_X_s32BEXVPosReq : Inport  Port=7  OutDataTypeStr=single
  yTmRefriVlvCtrl_B_BexvCalibReq : Inport  Port=8  OutDataTypeStr=boolean
  yTmRefriVlvCtrl_B_HpcBexvMovEnable : Inport  Port=9  OutDataTypeStr=boolean
  sTmRefriVlvCtrl_X_s32CEXVPosReq : Inport  Port=10  OutDataTypeStr=single
  yTmRefriVlvCtrl_B_CexvCalibReq : Inport  Port=11  OutDataTypeStr=boolean
  yTmRefriVlvCtrl_B_HpcCexvMovEnable : Inport  Port=12  OutDataTypeStr=boolean
  sTmColtVlvCtrl_D_u8HpcBctvRefDrvReq : Inport  Port=13  OutDataTypeStr=uint8
  sTmColtVlvCtrl_X_u8BctvPosReq : Inport  Port=14  OutDataTypeStr=uint8
  sTmColtVlvCtrl_D_u8HpcBcfvRefDrvReq : Inport  Port=15  OutDataTypeStr=uint8
  sTmDiag_D_u8VcEvLowSidePSnrSB : Inport  Port=16  OutDataTypeStr=uint8
  sTmDiag_D_u8VcEvLowSidePSnrOP : Inport  Port=17  OutDataTypeStr=uint8
  sTmDiag_D_u8VcEvHiSidePSnrOP : Inport  Port=18  OutDataTypeStr=uint8
  sTmDiag_D_u8VcEvHiSidePSnrSB : Inport  Port=19  OutDataTypeStr=uint8
  sTmDiag_D_u8VcEvHiSideTmpSnrSG : Inport  Port=20  OutDataTypeStr=uint8
  sTmDiag_D_u8VcEvHiSideTmpSnrOP : Inport  Port=21  OutDataTypeStr=uint8
  sTmDiag_D_u8VcEvBattCooltLvlLo : Inport  Port=22  OutDataTypeStr=uint8
  sTmDiag_D_u8VcEvSov1SB : Inport  Port=23  OutDataTypeStr=uint8
  sTmDiag_D_u8VcEvSov2SB : Inport  Port=24  OutDataTypeStr=uint8
  sTmDiag_D_u8VcEvSov3SB : Inport  Port=25  OutDataTypeStr=uint8
  sTmDiag_D_u8VcEvSov5SB : Inport  Port=26  OutDataTypeStr=uint8
  sTmDiag_D_u8VcEvSov4SB : Inport  Port=27  OutDataTypeStr=uint8
  sTmDiag_D_u8VcEvSBFan : Inport  Port=28  OutDataTypeStr=uint8
  sTmDiag_D_u8VcEvOPFan : Inport  Port=29  OutDataTypeStr=uint8
  sTmDiag_D_u8VcEvSGFan : Inport  Port=30  OutDataTypeStr=uint8
  sTmDiag_D_u8VcEvVolErrFan : Inport  Port=31  OutDataTypeStr=uint8
  sTmDiag_D_u8VcEvBlokFan : Inport  Port=32  OutDataTypeStr=uint8
  sTmDiag_D_u8VcEvCircutInteFlt : Inport  Port=33  OutDataTypeStr=uint8
  sTmDiag_D_u8VcEvHmPumpSB : Inport  Port=34  OutDataTypeStr=uint8
  sTmDiag_D_u8VcEvHmPumpOC : Inport  Port=35  OutDataTypeStr=uint8
  sTmDiag_D_u8HpmSov1Actv2FEnState : Inport  Port=36  OutDataTypeStr=uint8
  sTmDiag_D_u8HpmSov2Actv2FEnState : Inport  Port=37  OutDataTypeStr=uint8
  sTmDiag_D_u8HpmSov3Actv2FEnState : Inport  Port=38  OutDataTypeStr=uint8
  sTmDiag_D_u8FanPwm2FEnState : Inport  Port=39  OutDataTypeStr=uint8
  sTmDiag_D_u8BattCooltPmp2FEnState : Inport  Port=40  OutDataTypeStr=uint8
  sTmDiag_D_u8EmCooltPmp2FEnState : Inport  Port=41  OutDataTypeStr=uint8
  sTmDiag_D_u8PTCPumpSpd2FEnState : Inport  Port=42  OutDataTypeStr=uint8
  sTmDiag_D_u8EctvVlvMoveEna2FEnaState : Inport  Port=43  OutDataTypeStr=uint8
  sTmDiag_D_u8EctvVlvPos2FEnaState : Inport  Port=44  OutDataTypeStr=uint8
  sTmDiag_D_u8BctvVlvRef2FEnaState : Inport  Port=45  OutDataTypeStr=uint8
  sTmDiag_D_u8BctvVlvPos2FEnaState : Inport  Port=46  OutDataTypeStr=uint8
  sTmDiag_D_u8BcfvVlvRef2FEnaState : Inport  Port=47  OutDataTypeStr=uint8
  sTmDiag_D_u8BcfvVlvPos2FEnaState : Inport  Port=48  OutDataTypeStr=uint8
  sTmDiag_D_u8BexvCal2FEnaState : Inport  Port=49  OutDataTypeStr=uint8
  sTmDiag_D_u8BexvMoveEna2FEnaState : Inport  Port=50  OutDataTypeStr=uint8
  sTmDiag_D_u8BexvPosnReq2FEnaState : Inport  Port=51  OutDataTypeStr=uint8
  sTmDiag_D_u8CexvCal2FEnaState : Inport  Port=52  OutDataTypeStr=uint8
  sTmDiag_D_u8CexvMoveEna2FEnaState : Inport  Port=53  OutDataTypeStr=uint8
  sTmDiag_D_u8CexvPosnReq2FEnaState : Inport  Port=54  OutDataTypeStr=uint8
  sTmDiag_D_u8EexvCal2FEnaState : Inport  Port=55  OutDataTypeStr=uint8
  Conversion{,1..54} (55 alike) : SignalConversion  OverrideOpt=off
  TypeConvs : DataTypeConversion  OutDataTypeStr=uint8
  sTmOut_n_u16ElacCmprReq : Outport  OutDataTypeStr=uint16
  sTmOut_D_u8ElacCmprRelease : Outport  Port=2  OutDataTypeStr=uint8
  sTmOut_Pw_s32ElacCmprMax : Outport  Port=3  OutDataTypeStr=single
  sTmOut_X_s32EexvVlvPosReq : Outport  Port=4  OutDataTypeStr=single
  yTmOut_B_EexvPosnCalibReq : Outport  Port=5  OutDataTypeStr=boolean
  yTmOut_B_EexvPosnMovEnable : Outport  Port=6  OutDataTypeStr=boolean
  sTmOut_X_s32BexvVlvPosReq : Outport  Port=7  OutDataTypeStr=single
  yTmOut_B_BexvPosnCalibReq : Outport  Port=8  OutDataTypeStr=boolean
  yTmOut_B_BexvPosnMovEnable : Outport  Port=9  OutDataTypeStr=boolean
  sTmOut_X_s32CexvVlvPosReq : Outport  Port=10  OutDataTypeStr=single
  yTmOut_B_CexvPosnCalibReq : Outport  Port=11  OutDataTypeStr=boolean
  yTmOut_B_CexvPosnMovEnable : Outport  Port=12  OutDataTypeStr=boolean
  sTmOut_D_u8BctvVlvRefDrvReq : Outport  Port=13  OutDataTypeStr=uint8
  sTmOut_X_u8BctvVlvPosReq : Outport  Port=14  OutDataTypeStr=uint8
  sTmOut_D_u8BcfvVlvRefDrvReq : Outport  Port=15  OutDataTypeStr=uint8
  sTmOut_D_u8VcEvLowSidePSnrSB : Outport  Port=16  OutDataTypeStr=uint8
  sTmOut_D_u8VcEvLowSidePSnrOP : Outport  Port=17  OutDataTypeStr=uint8
  sTmOut_D_u8VcEvHiSidePSnrOP : Outport  Port=18  OutDataTypeStr=uint8
  sTmOut_D_u8VcEvHiSidePSnrSB : Outport  Port=19  OutDataTypeStr=uint8
  sTmOut_D_u8VcEvHiSideTmpSnrSG : Outport  Port=20  OutDataTypeStr=uint8
  sTmOut_D_u8VcEvHiSideTmpSnrOP : Outport  Port=21  OutDataTypeStr=uint8
  sTmOut_D_u8VcEvBattCooltLvlLo : Outport  Port=22  OutDataTypeStr=uint8
  sTmOut_D_u8VcEvSov1SB : Outport  Port=23  OutDataTypeStr=uint8
  sTmOut_D_u8VcEvSov2SB : Outport  Port=24  OutDataTypeStr=uint8
  sTmOut_D_u8VcEvSov3SB : Outport  Port=25  OutDataTypeStr=uint8
  sTmOut_D_u8VcEvSov5SB : Outport  Port=26  OutDataTypeStr=uint8
  sTmOut_D_u8VcEvSov4SB : Outport  Port=27  OutDataTypeStr=uint8
  sTmOut_D_u8VcEvSBFan : Outport  Port=28  OutDataTypeStr=uint8
  sTmOut_D_u8VcEvOPFan : Outport  Port=29  OutDataTypeStr=uint8
  sTmOut_D_u8VcEvSGFan : Outport  Port=30  OutDataTypeStr=uint8
  sTmOut_D_u8VcEvVolErrFan : Outport  Port=31  OutDataTypeStr=uint8
  sTmOut_D_u8VcEvBlokFan : Outport  Port=32  OutDataTypeStr=uint8
  sTmOut_D_u8VcEvCircutInteFlt : Outport  Port=33  OutDataTypeStr=uint8
  sTmOut_D_u8VcEvHmPumpSB : Outport  Port=34  OutDataTypeStr=uint8
  sTmOut_D_u8VcEvHmPumpOC : Outport  Port=35  OutDataTypeStr=uint8
  sTmOut_D_u8HpmSov1Actv2FEnState : Outport  Port=36  OutDataTypeStr=uint8
  sTmOut_D_u8HpmSov2Actv2FEnState : Outport  Port=37  OutDataTypeStr=uint8
  sTmOut_D_u8HpmSov3Actv2FEnState : Outport  Port=38  OutDataTypeStr=uint8
  sTmOut_D_u8FanPwm2FEnState : Outport  Port=39  OutDataTypeStr=uint8
  sTmOut_D_u8BattCooltPmp2FEnState : Outport  Port=40  OutDataTypeStr=uint8
  sTmOut_D_u8EmCooltPmp2FEnState : Outport  Port=41  OutDataTypeStr=uint8
  sTmOut_D_u8PTCPumpSpd2FEnState : Outport  Port=42  OutDataTypeStr=uint8
  sTmOut_D_u8EctvVlvMoveEna2FEnaState : Outport  Port=43  OutDataTypeStr=uint8
  sTmOut_D_u8EctvVlvPos2FEnaState : Outport  Port=44  OutDataTypeStr=uint8
  sTmOut_D_u8BctvVlvRef2FEnaState : Outport  Port=45  OutDataTypeStr=uint8
  sTmOut_D_u8BctvVlvPos2FEnaState : Outport  Port=46  OutDataTypeStr=uint8
  sTmOut_D_u8BcfvVlvRef2FEnaState : Outport  Port=47  OutDataTypeStr=uint8
  sTmOut_D_u8BcfvVlvPos2FEnaState : Outport  Port=48  OutDataTypeStr=uint8
  sTmOut_D_u8BexvCal2FEnaState : Outport  Port=49  OutDataTypeStr=uint8
  sTmOut_D_u8BexvMoveEna2FEnaState : Outport  Port=50  OutDataTypeStr=uint8
  sTmOut_D_u8BexvPosnReq2FEnaState : Outport  Port=51  OutDataTypeStr=uint8
  sTmOut_D_u8CexvCal2FEnaState : Outport  Port=52  OutDataTypeStr=uint8
  sTmOut_D_u8CexvMoveEna2FEnaState : Outport  Port=53  OutDataTypeStr=uint8
  sTmOut_D_u8CexvPosnReq2FEnaState : Outport  Port=54  OutDataTypeStr=uint8
  sTmOut_D_u8EexvCal2FEnaState : Outport  Port=55  OutDataTypeStr=uint8
  wires:
  sTmComprCtrl_n_u16CompRpmReq/1 -> Conversion/1  "sTmComprCtrl_n_u16CompRpmReq"
  Conversion/1 -> sTmOut_n_u16ElacCmprReq/1  "sTmOut_n_u16ElacCmprReq"
  yTmComprCtrl_B_CompOnReq/1 -> Conversion1/1  "yTmComprCtrl_B_CompOnReq"
  Conversion1/1 -> TypeConvs/1
  TypeConvs/1 -> sTmOut_D_u8ElacCmprRelease/1  "sTmOut_D_u8ElacCmprRelease"
  sTmEnergyMgr_Pw_s32AcCmprPwrLim/1 -> Conversion2/1  "sTmEnergyMgr_Pw_s32AcCmprPwrLim"
  Conversion2/1 -> sTmOut_Pw_s32ElacCmprMax/1  "sTmOut_Pw_s32ElacCmprMax"
  sTmRefriVlvCtrl_X_s32EEXVPosReq/1 -> Conversion3/1  "sTmRefriVlvCtrl_X_s32EEXVPosReq"
  Conversion3/1 -> sTmOut_X_s32EexvVlvPosReq/1  "sTmOut_X_s32EexvVlvPosReq"
  yTmRefriVlvCtrl_B_EexvCalibReq/1 -> Conversion4/1  "yTmRefriVlvCtrl_B_EexvCalibReq"
  Conversion4/1 -> yTmOut_B_EexvPosnCalibReq/1  "yTmOut_B_EexvPosnCalibReq"
  yTmRefriVlvCtrl_B_HpcEexvMovEnable/1 -> Conversion5/1  "yTmRefriVlvCtrl_B_HpcEexvMovEnable"
  Conversion5/1 -> yTmOut_B_EexvPosnMovEnable/1  "yTmOut_B_EexvPosnMovEnable"
  sTmRefriVlvCtrl_X_s32BEXVPosReq/1 -> Conversion6/1  "sTmRefriVlvCtrl_X_s32BEXVPosReq"
  Conversion6/1 -> sTmOut_X_s32BexvVlvPosReq/1  "sTmOut_X_s32BexvVlvPosReq"
  yTmRefriVlvCtrl_B_BexvCalibReq/1 -> Conversion7/1  "yTmRefriVlvCtrl_B_BexvCalibReq"
  Conversion7/1 -> yTmOut_B_BexvPosnCalibReq/1  "yTmOut_B_BexvPosnCalibReq"
  yTmRefriVlvCtrl_B_HpcBexvMovEnable/1 -> Conversion8/1  "yTmRefriVlvCtrl_B_HpcBexvMovEnable"
  Conversion8/1 -> yTmOut_B_BexvPosnMovEnable/1  "yTmOut_B_BexvPosnMovEnable"
  sTmRefriVlvCtrl_X_s32CEXVPosReq/1 -> Conversion9/1  "sTmRefriVlvCtrl_X_s32CEXVPosReq"
  Conversion9/1 -> sTmOut_X_s32CexvVlvPosReq/1  "sTmOut_X_s32CexvVlvPosReq"
  yTmRefriVlvCtrl_B_CexvCalibReq/1 -> Conversion10/1  "yTmRefriVlvCtrl_B_CexvCalibReq"
  Conversion10/1 -> yTmOut_B_CexvPosnCalibReq/1  "yTmOut_B_CexvPosnCalibReq"
  yTmRefriVlvCtrl_B_HpcCexvMovEnable/1 -> Conversion11/1  "yTmRefriVlvCtrl_B_HpcCexvMovEnable"
  Conversion11/1 -> yTmOut_B_CexvPosnMovEnable/1  "yTmOut_B_CexvPosnMovEnable"
  sTmColtVlvCtrl_D_u8HpcBctvRefDrvReq/1 -> Conversion12/1  "sTmColtVlvCtrl_D_u8HpcBctvRefDrvReq"
  Conversion12/1 -> sTmOut_D_u8BctvVlvRefDrvReq/1  "sTmOut_D_u8BctvVlvRefDrvReq"
  sTmColtVlvCtrl_X_u8BctvPosReq/1 -> Conversion13/1  "sTmColtVlvCtrl_X_u8BctvPosReq"
  Conversion13/1 -> sTmOut_X_u8BctvVlvPosReq/1  "sTmOut_X_u8BctvVlvPosReq"
  sTmColtVlvCtrl_D_u8HpcBcfvRefDrvReq/1 -> Conversion14/1  "sTmColtVlvCtrl_D_u8HpcBcfvRefDrvReq"
  Conversion14/1 -> sTmOut_D_u8BcfvVlvRefDrvReq/1  "sTmOut_D_u8BcfvVlvRefDrvReq"
  sTmDiag_D_u8VcEvLowSidePSnrSB/1 -> Conversion15/1  "sTmDiag_D_u8VcEvLowSidePSnrSB"
  Conversion15/1 -> sTmOut_D_u8VcEvLowSidePSnrSB/1  "sTmOut_D_u8VcEvLowSidePSnrSB"
  sTmDiag_D_u8VcEvLowSidePSnrOP/1 -> Conversion16/1  "sTmDiag_D_u8VcEvLowSidePSnrOP"
  Conversion16/1 -> sTmOut_D_u8VcEvLowSidePSnrOP/1  "sTmOut_D_u8VcEvLowSidePSnrOP"
  sTmDiag_D_u8VcEvHiSidePSnrOP/1 -> Conversion17/1  "sTmDiag_D_u8VcEvHiSidePSnrOP"
  Conversion17/1 -> sTmOut_D_u8VcEvHiSidePSnrOP/1  "sTmOut_D_u8VcEvHiSidePSnrOP"
  sTmDiag_D_u8VcEvHiSidePSnrSB/1 -> Conversion18/1  "sTmDiag_D_u8VcEvHiSidePSnrSB"
  Conversion18/1 -> sTmOut_D_u8VcEvHiSidePSnrSB/1  "sTmOut_D_u8VcEvHiSidePSnrSB"
  sTmDiag_D_u8VcEvHiSideTmpSnrSG/1 -> Conversion19/1  "sTmDiag_D_u8VcEvHiSideTmpSnrSG"
  Conversion19/1 -> sTmOut_D_u8VcEvHiSideTmpSnrSG/1  "sTmOut_D_u8VcEvHiSideTmpSnrSG"
  sTmDiag_D_u8VcEvHiSideTmpSnrOP/1 -> Conversion20/1  "sTmDiag_D_u8VcEvHiSideTmpSnrOP"
  Conversion20/1 -> sTmOut_D_u8VcEvHiSideTmpSnrOP/1  "sTmOut_D_u8VcEvHiSideTmpSnrOP"
  sTmDiag_D_u8VcEvBattCooltLvlLo/1 -> Conversion21/1  "sTmDiag_D_u8VcEvBattCooltLvlLo"
  Conversion21/1 -> sTmOut_D_u8VcEvBattCooltLvlLo/1  "sTmOut_D_u8VcEvBattCooltLvlLo"
  sTmDiag_D_u8VcEvSov1SB/1 -> Conversion22/1  "sTmDiag_D_u8VcEvSov1SB"
  Conversion22/1 -> sTmOut_D_u8VcEvSov1SB/1  "sTmOut_D_u8VcEvSov1SB"
  sTmDiag_D_u8VcEvSov2SB/1 -> Conversion23/1  "sTmDiag_D_u8VcEvSov2SB"
  Conversion23/1 -> sTmOut_D_u8VcEvSov2SB/1  "sTmOut_D_u8VcEvSov2SB"
  sTmDiag_D_u8VcEvSov3SB/1 -> Conversion24/1  "sTmDiag_D_u8VcEvSov3SB"
  Conversion24/1 -> sTmOut_D_u8VcEvSov3SB/1  "sTmOut_D_u8VcEvSov3SB"
  sTmDiag_D_u8VcEvSov5SB/1 -> Conversion25/1  "sTmDiag_D_u8VcEvSov5SB"
  Conversion25/1 -> sTmOut_D_u8VcEvSov5SB/1  "sTmOut_D_u8VcEvSov5SB"
  sTmDiag_D_u8VcEvSov4SB/1 -> Conversion26/1  "sTmDiag_D_u8VcEvSov4SB"
  Conversion26/1 -> sTmOut_D_u8VcEvSov4SB/1  "sTmOut_D_u8VcEvSov4SB"
  sTmDiag_D_u8VcEvSBFan/1 -> Conversion27/1  "sTmDiag_D_u8VcEvSBFan"
  Conversion27/1 -> sTmOut_D_u8VcEvSBFan/1  "sTmOut_D_u8VcEvSBFan"
  sTmDiag_D_u8VcEvOPFan/1 -> Conversion28/1  "sTmDiag_D_u8VcEvOPFan"
  Conversion28/1 -> sTmOut_D_u8VcEvOPFan/1  "sTmOut_D_u8VcEvOPFan"
  sTmDiag_D_u8VcEvSGFan/1 -> Conversion29/1  "sTmDiag_D_u8VcEvSGFan"
  Conversion29/1 -> sTmOut_D_u8VcEvSGFan/1  "sTmOut_D_u8VcEvSGFan"
  sTmDiag_D_u8VcEvVolErrFan/1 -> Conversion30/1  "sTmDiag_D_u8VcEvVolErrFan"
  Conversion30/1 -> sTmOut_D_u8VcEvVolErrFan/1  "sTmOut_D_u8VcEvVolErrFan"
  sTmDiag_D_u8VcEvBlokFan/1 -> Conversion31/1  "sTmDiag_D_u8VcEvBlokFan"
  Conversion31/1 -> sTmOut_D_u8VcEvBlokFan/1  "sTmOut_D_u8VcEvBlokFan"
  sTmDiag_D_u8VcEvCircutInteFlt/1 -> Conversion32/1  "sTmDiag_D_u8VcEvCircutInteFlt"
  Conversion32/1 -> sTmOut_D_u8VcEvCircutInteFlt/1  "sTmOut_D_u8VcEvCircutInteFlt"
  sTmDiag_D_u8VcEvHmPumpSB/1 -> Conversion33/1  "sTmDiag_D_u8VcEvHmPumpSB"
  Conversion33/1 -> sTmOut_D_u8VcEvHmPumpSB/1  "sTmOut_D_u8VcEvHmPumpSB"
  sTmDiag_D_u8VcEvHmPumpOC/1 -> Conversion34/1  "sTmDiag_D_u8VcEvHmPumpOC"
  Conversion34/1 -> sTmOut_D_u8VcEvHmPumpOC/1  "sTmOut_D_u8VcEvHmPumpOC"
  sTmDiag_D_u8HpmSov1Actv2FEnState/1 -> Conversion35/1  "sTmDiag_D_u8HpmSov1Actv2FEnState"
  Conversion35/1 -> sTmOut_D_u8HpmSov1Actv2FEnState/1  "sTmOut_D_u8HpmSov1Actv2FEnState"
  sTmDiag_D_u8HpmSov2Actv2FEnState/1 -> Conversion36/1  "sTmDiag_D_u8HpmSov2Actv2FEnState"
  Conversion36/1 -> sTmOut_D_u8HpmSov2Actv2FEnState/1  "sTmOut_D_u8HpmSov2Actv2FEnState"
  sTmDiag_D_u8HpmSov3Actv2FEnState/1 -> Conversion37/1  "sTmDiag_D_u8HpmSov3Actv2FEnState"
  Conversion37/1 -> sTmOut_D_u8HpmSov3Actv2FEnState/1  "sTmOut_D_u8HpmSov3Actv2FEnState"
  sTmDiag_D_u8FanPwm2FEnState/1 -> Conversion38/1  "sTmDiag_D_u8FanPwm2FEnState"
  Conversion38/1 -> sTmOut_D_u8FanPwm2FEnState/1  "sTmOut_D_u8FanPwm2FEnState"
  sTmDiag_D_u8BattCooltPmp2FEnState/1 -> Conversion39/1  "sTmDiag_D_u8BattCooltPmp2FEnState"
  Conversion39/1 -> sTmOut_D_u8BattCooltPmp2FEnState/1  "sTmOut_D_u8BattCooltPmp2FEnState"
  sTmDiag_D_u8EmCooltPmp2FEnState/1 -> Conversion40/1  "sTmDiag_D_u8EmCooltPmp2FEnState"
  Conversion40/1 -> sTmOut_D_u8EmCooltPmp2FEnState/1  "sTmOut_D_u8EmCooltPmp2FEnState"
  sTmDiag_D_u8PTCPumpSpd2FEnState/1 -> Conversion41/1  "sTmDiag_D_u8PTCPumpSpd2FEnState"
  Conversion41/1 -> sTmOut_D_u8PTCPumpSpd2FEnState/1  "sTmOut_D_u8PTCPumpSpd2FEnState"
  sTmDiag_D_u8EctvVlvMoveEna2FEnaState/1 -> Conversion42/1  "sTmDiag_D_u8EctvVlvMoveEna2FEnaState"
  Conversion42/1 -> sTmOut_D_u8EctvVlvMoveEna2FEnaState/1  "sTmOut_D_u8EctvVlvMoveEna2FEnaState"
  sTmDiag_D_u8EctvVlvPos2FEnaState/1 -> Conversion43/1  "sTmDiag_D_u8EctvVlvPos2FEnaState"
  Conversion43/1 -> sTmOut_D_u8EctvVlvPos2FEnaState/1  "sTmOut_D_u8EctvVlvPos2FEnaState"
  sTmDiag_D_u8BctvVlvRef2FEnaState/1 -> Conversion44/1  "sTmDiag_D_u8BctvVlvRef2FEnaState"
  Conversion44/1 -> sTmOut_D_u8BctvVlvRef2FEnaState/1  "sTmOut_D_u8BctvVlvRef2FEnaState"
  sTmDiag_D_u8BctvVlvPos2FEnaState/1 -> Conversion45/1  "sTmDiag_D_u8BctvVlvPos2FEnaState"
  Conversion45/1 -> sTmOut_D_u8BctvVlvPos2FEnaState/1  "sTmOut_D_u8BctvVlvPos2FEnaState"
  sTmDiag_D_u8BcfvVlvRef2FEnaState/1 -> Conversion46/1  "sTmDiag_D_u8BcfvVlvRef2FEnaState"
  Conversion46/1 -> sTmOut_D_u8BcfvVlvRef2FEnaState/1  "sTmOut_D_u8BcfvVlvRef2FEnaState"
  sTmDiag_D_u8BcfvVlvPos2FEnaState/1 -> Conversion47/1  "sTmDiag_D_u8BcfvVlvPos2FEnaState"
  Conversion47/1 -> sTmOut_D_u8BcfvVlvPos2FEnaState/1  "sTmOut_D_u8BcfvVlvPos2FEnaState"
  sTmDiag_D_u8BexvCal2FEnaState/1 -> Conversion48/1  "sTmDiag_D_u8BexvCal2FEnaState"
  Conversion48/1 -> sTmOut_D_u8BexvCal2FEnaState/1  "sTmOut_D_u8BexvCal2FEnaState"
  sTmDiag_D_u8BexvMoveEna2FEnaState/1 -> Conversion49/1  "sTmDiag_D_u8BexvMoveEna2FEnaState"
  Conversion49/1 -> sTmOut_D_u8BexvMoveEna2FEnaState/1  "sTmOut_D_u8BexvMoveEna2FEnaState"
  sTmDiag_D_u8BexvPosnReq2FEnaState/1 -> Conversion50/1  "sTmDiag_D_u8BexvPosnReq2FEnaState"
  Conversion50/1 -> sTmOut_D_u8BexvPosnReq2FEnaState/1  "sTmOut_D_u8BexvPosnReq2FEnaState"
  sTmDiag_D_u8CexvCal2FEnaState/1 -> Conversion51/1  "sTmDiag_D_u8CexvCal2FEnaState"
  Conversion51/1 -> sTmOut_D_u8CexvCal2FEnaState/1  "sTmOut_D_u8CexvCal2FEnaState"
  sTmDiag_D_u8CexvMoveEna2FEnaState/1 -> Conversion52/1  "sTmDiag_D_u8CexvMoveEna2FEnaState"
  Conversion52/1 -> sTmOut_D_u8CexvMoveEna2FEnaState/1  "sTmOut_D_u8CexvMoveEna2FEnaState"
  sTmDiag_D_u8CexvPosnReq2FEnaState/1 -> Conversion53/1  "sTmDiag_D_u8CexvPosnReq2FEnaState"
  Conversion53/1 -> sTmOut_D_u8CexvPosnReq2FEnaState/1  "sTmOut_D_u8CexvPosnReq2FEnaState"
  sTmDiag_D_u8EexvCal2FEnaState/1 -> Conversion54/1  "sTmDiag_D_u8EexvCal2FEnaState"
  Conversion54/1 -> sTmOut_D_u8EexvCal2FEnaState/1  "sTmOut_D_u8EexvCal2FEnaState"

== system ScriptDemo/Create/createBus/createBusGoto ==
  After : Subsystem
  Before : Subsystem

== system ScriptDemo/Create/createBus/createBusPort ==
  After : Subsystem
  Before : Subsystem

== system ScriptDemo/Create/createDebug/After ==
  After : Subsystem
  sTmRefriVlvCtrl_X_s32CEXVPosReq : Outport  OutDataTypeStr=single
  sTmRefriVlvCtrl_X_s32EEXVPosReq : Outport  Port=2  OutDataTypeStr=single
  sTmRefriVlvCtrl_X_s32BEXVPosReq : Outport  Port=3  OutDataTypeStr=single
  yTmRefriVlvCtrl_B_HpcCexvMovEnable : Outport  Port=4  OutDataTypeStr=boolean
  sTmRefriVlvCtrl_Z_u8CEXVInitState : Outport  Port=5  OutDataTypeStr=uint8
  yTmRefriVlvCtrl_B_CexvCalibReq : Outport  Port=6  OutDataTypeStr=boolean
  yTmRefriVlvCtrl_B_HpcEexvMovEnable : Outport  Port=7  OutDataTypeStr=boolean
  sTmRefriVlvCtrl_Z_u8EEXVInitState : Outport  Port=8  OutDataTypeStr=uint8
  yTmRefriVlvCtrl_B_EexvCalibReq : Outport  Port=9  OutDataTypeStr=boolean
  yTmRefriVlvCtrl_B_HpcBexvMovEnable : Outport  Port=10  OutDataTypeStr=boolean
  sTmRefriVlvCtrl_Z_u8BEXVInitState : Outport  Port=11  OutDataTypeStr=uint8
  yTmRefriVlvCtrl_B_BexvCalibReq : Outport  Port=12  OutDataTypeStr=boolean
  sTmRefriVlvCtrl_X_s32SM3BexvMaxPos : Outport  Port=13  OutDataTypeStr=single
  yTmRefriVlvCtrl_B_EvapBattTLimBexvEna : Outport  Port=14  OutDataTypeStr=boolean
  sTmRefriVlvCtrl_D_u8EexvRefriSwitchSt : Outport  Port=15  OutDataTypeStr=uint8
  sTmRefriVlvCtrl_D_u8CexvRefriSwitchSt : Outport  Port=16  OutDataTypeStr=uint8
  sTmRefriVlvCtrl_D_u8BexvRefriSwitchSt : Outport  Port=17  OutDataTypeStr=uint8
  wires:
  After/11(sTmRefriVlvCtrl_Z_u8BEXVInitState) -> sTmRefriVlvCtrl_Z_u8BEXVInitState/1
  [sTmRefriVlvCtrl_D_u8EexvRefriSwitchSt] -> After/15(sTmRefriVlvCtrl_D_u8EexvRefriSwitchStDbgin)
  After/2(sTmRefriVlvCtrl_X_s32EEXVPosReq) -> sTmRefriVlvCtrl_X_s32EEXVPosReq/1
  After/14(yTmRefriVlvCtrl_B_EvapBattTLimBexvEna) -> yTmRefriVlvCtrl_B_EvapBattTLimBexvEna/1
  [sTmRefriVlvCtrl_X_s32EEXVPosReq] -> After/2(sTmRefriVlvCtrl_X_s32EEXVPosReqDbgin)
  After/5(sTmRefriVlvCtrl_Z_u8CEXVInitState) -> sTmRefriVlvCtrl_Z_u8CEXVInitState/1
  [yTmRefriVlvCtrl_B_HpcBexvMovEnable] -> After/10(yTmRefriVlvCtrl_B_HpcBexvMovEnableDbgin)
  [sTmRefriVlvCtrl_X_s32SM3BexvMaxPos] -> After/13(sTmRefriVlvCtrl_X_s32SM3BexvMaxPosDbgin)
  After/3(sTmRefriVlvCtrl_X_s32BEXVPosReq) -> sTmRefriVlvCtrl_X_s32BEXVPosReq/1
  [yTmRefriVlvCtrl_B_BexvCalibReq] -> After/12(yTmRefriVlvCtrl_B_BexvCalibReqDbgin)
  [sTmRefriVlvCtrl_D_u8BexvRefriSwitchSt] -> After/17(sTmRefriVlvCtrl_D_u8BexvRefriSwitchStDbgin)
  After/12(yTmRefriVlvCtrl_B_BexvCalibReq) -> yTmRefriVlvCtrl_B_BexvCalibReq/1
  [sTmRefriVlvCtrl_D_u8CexvRefriSwitchSt] -> After/16(sTmRefriVlvCtrl_D_u8CexvRefriSwitchStDbgin)
  [sTmRefriVlvCtrl_X_s32CEXVPosReq] -> After/1(sTmRefriVlvCtrl_X_s32CEXVPosReqDbgin)
  [sTmRefriVlvCtrl_Z_u8BEXVInitState] -> After/11(sTmRefriVlvCtrl_Z_u8BEXVInitStateDbgin)
  After/1(sTmRefriVlvCtrl_X_s32CEXVPosReq) -> sTmRefriVlvCtrl_X_s32CEXVPosReq/1
  [yTmRefriVlvCtrl_B_HpcCexvMovEnable] -> After/4(yTmRefriVlvCtrl_B_HpcCexvMovEnableDbgin)
  [yTmRefriVlvCtrl_B_CexvCalibReq] -> After/6(yTmRefriVlvCtrl_B_CexvCalibReqDbgin)
  After/8(sTmRefriVlvCtrl_Z_u8EEXVInitState) -> sTmRefriVlvCtrl_Z_u8EEXVInitState/1
  [yTmRefriVlvCtrl_B_HpcEexvMovEnable] -> After/7(yTmRefriVlvCtrl_B_HpcEexvMovEnableDbgin)
  [yTmRefriVlvCtrl_B_EexvCalibReq] -> After/9(yTmRefriVlvCtrl_B_EexvCalibReqDbgin)
  After/16(sTmRefriVlvCtrl_D_u8CexvRefriSwitchSt) -> sTmRefriVlvCtrl_D_u8CexvRefriSwitchSt/1
  After/6(yTmRefriVlvCtrl_B_CexvCalibReq) -> yTmRefriVlvCtrl_B_CexvCalibReq/1
  After/10(yTmRefriVlvCtrl_B_HpcBexvMovEnable) -> yTmRefriVlvCtrl_B_HpcBexvMovEnable/1
  After/13(sTmRefriVlvCtrl_X_s32SM3BexvMaxPos) -> sTmRefriVlvCtrl_X_s32SM3BexvMaxPos/1
  After/9(yTmRefriVlvCtrl_B_EexvCalibReq) -> yTmRefriVlvCtrl_B_EexvCalibReq/1
  After/4(yTmRefriVlvCtrl_B_HpcCexvMovEnable) -> yTmRefriVlvCtrl_B_HpcCexvMovEnable/1
  After/15(sTmRefriVlvCtrl_D_u8EexvRefriSwitchSt) -> sTmRefriVlvCtrl_D_u8EexvRefriSwitchSt/1
  [sTmRefriVlvCtrl_X_s32BEXVPosReq] -> After/3(sTmRefriVlvCtrl_X_s32BEXVPosReqDbgin)
  After/7(yTmRefriVlvCtrl_B_HpcEexvMovEnable) -> yTmRefriVlvCtrl_B_HpcEexvMovEnable/1
  [sTmRefriVlvCtrl_Z_u8EEXVInitState] -> After/8(sTmRefriVlvCtrl_Z_u8EEXVInitStateDbgin)
  After/17(sTmRefriVlvCtrl_D_u8BexvRefriSwitchSt) -> sTmRefriVlvCtrl_D_u8BexvRefriSwitchSt/1
  [sTmRefriVlvCtrl_Z_u8CEXVInitState] -> After/5(sTmRefriVlvCtrl_Z_u8CEXVInitStateDbgin)
  [yTmRefriVlvCtrl_B_EvapBattTLimBexvEna] -> After/14(yTmRefriVlvCtrl_B_EvapBattTLimBexvEnaDbgin)

== system ScriptDemo/Create/createDebug/After1 ==
  note: % 目的: 为输出端口创建debug 及对应的输入模块
      | [cnt] = createDebug(gcs,'NameInType','findLoc')
  rLocModeName_X_s32CEXVPosReq : Inport  OutDataTypeStr=single
  ScriptDemo_X_s32EEXVPosReq : Inport  Port=2  OutDataTypeStr=single
  rLocModeName_X_s32BEXVPosReq : Inport  Port=3  OutDataTypeStr=single
  OutDebug : PCMULib/Interface/OutdebugRvs  SWI=cTmRefriVlvCtrl_X_s32CEXVPosReq_sw  DBI=cTmRefriVlvCtrl_X_s32CEXVPosReq_db
      settings: SourceProductName=PCMULib
  OutDebug1 : PCMULib/Interface/OutdebugRvs  SWI=cTmRefriVlvCtrl_X_s32EEXVPosReq_sw  DBI=cTmRefriVlvCtrl_X_s32EEXVPosReq_db
      settings: SourceProductName=PCMULib
  OutDebug2 : PCMULib/Interface/OutdebugRvs  SWI=cTmRefriVlvCtrl_X_s32BEXVPosReq_sw  DBI=cTmRefriVlvCtrl_X_s32BEXVPosReq_db
      settings: SourceProductName=PCMULib
  sTmRefriVlvCtrl_X_s32CEXVPosReq : Outport  OutDataTypeStr=single
  sTmRefriVlvCtrl_X_s32EEXVPosReq : Outport  Port=2  OutDataTypeStr=single
  sTmRefriVlvCtrl_X_s32BEXVPosReq : Outport  Port=3  OutDataTypeStr=single
  wires:
  rLocModeName_X_s32CEXVPosReq/1 -> OutDebug/1
  OutDebug/1 -> sTmRefriVlvCtrl_X_s32CEXVPosReq/1
  ScriptDemo_X_s32EEXVPosReq/1 -> OutDebug1/1
  OutDebug1/1 -> sTmRefriVlvCtrl_X_s32EEXVPosReq/1
  rLocModeName_X_s32BEXVPosReq/1 -> OutDebug2/1
  OutDebug2/1 -> sTmRefriVlvCtrl_X_s32BEXVPosReq/1

== system ScriptDemo/Create/createDebug/Before ==
  note: % 目的: 为输出端口创建debug 及对应的输入模块
      | [cnt] = createDebug(gcs)
  sTmRefriVlvCtrl_X_s32CEXVPosReq : Outport  OutDataTypeStr=single
  sTmRefriVlvCtrl_X_s32EEXVPosReq : Outport  Port=2  OutDataTypeStr=single
  sTmRefriVlvCtrl_X_s32BEXVPosReq : Outport  Port=3  OutDataTypeStr=single
  yTmRefriVlvCtrl_B_HpcCexvMovEnable : Outport  Port=4  OutDataTypeStr=boolean
  sTmRefriVlvCtrl_Z_u8CEXVInitState : Outport  Port=5  OutDataTypeStr=uint8
  yTmRefriVlvCtrl_B_CexvCalibReq : Outport  Port=6  OutDataTypeStr=boolean
  yTmRefriVlvCtrl_B_HpcEexvMovEnable : Outport  Port=7  OutDataTypeStr=boolean
  sTmRefriVlvCtrl_Z_u8EEXVInitState : Outport  Port=8  OutDataTypeStr=uint8
  yTmRefriVlvCtrl_B_EexvCalibReq : Outport  Port=9  OutDataTypeStr=boolean
  yTmRefriVlvCtrl_B_HpcBexvMovEnable : Outport  Port=10  OutDataTypeStr=boolean
  sTmRefriVlvCtrl_Z_u8BEXVInitState : Outport  Port=11  OutDataTypeStr=uint8
  yTmRefriVlvCtrl_B_BexvCalibReq : Outport  Port=12  OutDataTypeStr=boolean
  sTmRefriVlvCtrl_X_s32SM3BexvMaxPos : Outport  Port=13  OutDataTypeStr=single
  yTmRefriVlvCtrl_B_EvapBattTLimBexvEna : Outport  Port=14  OutDataTypeStr=boolean
  sTmRefriVlvCtrl_D_u8EexvRefriSwitchSt : Outport  Port=15  OutDataTypeStr=uint8
  sTmRefriVlvCtrl_D_u8CexvRefriSwitchSt : Outport  Port=16  OutDataTypeStr=uint8
  sTmRefriVlvCtrl_D_u8BexvRefriSwitchSt : Outport  Port=17  OutDataTypeStr=uint8

== system ScriptDemo/Create/createDebug/Before1 ==
  note: % 目的: 为输出端口创建debug 及对应的输入模块
      | [cnt] = createDebug(gcs,'NameInType','findLoc')
  sTmRefriVlvCtrl_X_s32CEXVPosReq : Outport  OutDataTypeStr=single
  sTmRefriVlvCtrl_X_s32EEXVPosReq : Outport  Port=2  OutDataTypeStr=single
  sTmRefriVlvCtrl_X_s32BEXVPosReq : Outport  Port=3  OutDataTypeStr=single
